simulink model "robotarm_part_both"  (R2018b)
settings: Solver=FixedStepAuto  StartTime=0.0  StopTime=options.T_train-options.dt  RelTol=1e-3  AbsTol=1e-6
undefined symbols (not defined in the file or in its folder): options
libraries: neural x132, simulink x4
(part 2 of 6)

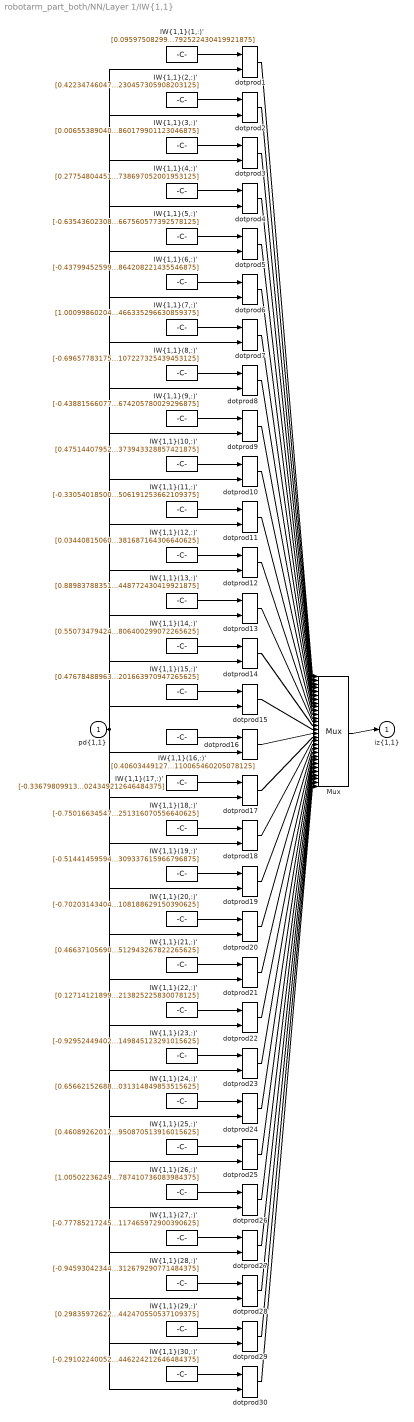
== system robotarm_part_both/NN/Layer 1/IW{1,1} ==
  "pd{1,1}" : Inport  PortDimensions=10
      mask Display: e = 0.06;c1 = [120 230 180]/255;c2 = ([120 230 180]+0)/(256+128);c3 = ([120 230 180]+128)/(256+128);patch([0 1 1 0],[0 0 1 1],c1);patch([0 1 1 1-e 1-e 0+e],[0 0 1 1-e 0+e 0+e],c2);patch([0 0 1 1-e 0+e 0+e],[0 1 1 1-e 1-e 0+e],c3);plot([0 1 1 0 0],[0 0 1 1 0]);
  "IW{1,1}(1,:)'" : Constant  Value=[0.09597508299962474731525929882991476915776729583740234375;0.1005968170649829962481902612125850282609462738037109375;-0.55045262317495780024501073057763278484344482421875;-0.5647944454818947246366178660537116229534149169921875;0.18118548745802998123366478466778062283992767333984375;0.9302020854734853738676747525460086762905120849609375;0.33129531414507751296838478083373047411441802978515625;1.2080937875825370486637666544993408024311065673828125;-0.303614801234934839069268264211132191121578216552734375;-0.64616365051114577067181699021602980792522430419921875]
      mask Display: e = 0.06;c1 = [120 150 230]/255;c2 = ([120 150 230]+0)/383;c3 = ([120 150 230]+128)/383;patch([0 1 1 0],[0 0 1 1],c1);patch([0 1 1 1-e 1-e 0+e],[0 0 1 1-e 0+e 0+e],c2);patch([0 0 1 1-e 0+e 0+e],[0 1 1 1-e 1-e 0+e],c3);plot([0 1 1 0 0],[0 0 1 1 0]);disp('Weights');
  "IW{1,1}(10,:)'" : Constant  Value=[0.47514407952864823325711540746851824223995208740234375;-0.5065631999531381435275534386164508759975433349609375;0.423535188943548301931940613940241746604442596435546875;0.58875725936849587771604319641483016312122344970703125;0.07117432075978487315826015446873498149216175079345703125;-0.5875257273326657259104877084610052406787872314453125;-1.1175178395749139070858291233889758586883544921875;-0.6724331101001104205039382577524520456790924072265625;0.1606137196925800647573367996301385574042797088623046875;-0.0059917862738066256234059636653910274617373943328857421875]
      mask Display: e = 0.06;c1 = [120 150 230]/255;c2 = ([120 150 230]+0)/383;c3 = ([120 150 230]+128)/383;patch([0 1 1 0],[0 0 1 1],c1);patch([0 1 1 1-e 1-e 0+e],[0 0 1 1-e 0+e 0+e],c2);patch([0 0 1 1-e 0+e 0+e],[0 1 1 1-e 1-e 0+e],c3);plot([0 1 1 0 0],[0 0 1 1 0]);disp('Weights');
  "IW{1,1}(11,:)'" : Constant  Value=[-0.330540185002522968193972019435022957623004913330078125;-0.5853737960314406851836110945441760122776031494140625;-0.373973670570021343717570516673731617629528045654296875;-0.457347659514774462774511221141437999904155731201171875;-0.41561353090748831551337616474484093487262725830078125;0.51656871771152046424191439655260182917118072509765625;0.65290213175343636553549231393844820559024810791015625;-0.91601082511943066055692952431854791939258575439453125;-0.414078886006279012210740120281116105616092681884765625;-0.64754463829876518499162330044782720506191253662109375]
      mask Display: e = 0.06;c1 = [120 150 230]/255;c2 = ([120 150 230]+0)/383;c3 = ([120 150 230]+128)/383;patch([0 1 1 0],[0 0 1 1],c1);patch([0 1 1 1-e 1-e 0+e],[0 0 1 1-e 0+e 0+e],c2);patch([0 0 1 1-e 0+e 0+e],[0 1 1 1-e 1-e 0+e],c3);plot([0 1 1 0 0],[0 0 1 1 0]);disp('Weights');
  "IW{1,1}(12,:)'" : Constant  Value=[0.03440815060161195315657778337481431663036346435546875;-0.550528645065602173502838923013769090175628662109375;0.10571613935137315343215647089891717769205570220947265625;-0.50746669530979826578942493142676539719104766845703125;1.216730766600212287897875285125337541103363037109375;0.1123742853737608182740359552553854882717132568359375;-0.66521689864983069018222749946289695799350738525390625;-0.8226026955605025836604227151838131248950958251953125;0.09635653093671248115015259827487170696258544921875;0.92693103311651869891107935472973622381687164306640625]
      mask Display: e = 0.06;c1 = [120 150 230]/255;c2 = ([120 150 230]+0)/383;c3 = ([120 150 230]+128)/383;patch([0 1 1 0],[0 0 1 1],c1);patch([0 1 1 1-e 1-e 0+e],[0 0 1 1-e 0+e 0+e],c2);patch([0 0 1 1-e 0+e 0+e],[0 1 1 1-e 1-e 0+e],c3);plot([0 1 1 0 0],[0 0 1 1 0]);disp('Weights');
  "IW{1,1}(13,:)'" : Constant  Value=[0.889837883519465577819573809392750263214111328125;-0.8578294294074966241936408550827763974666595458984375;-0.50271543951528119276161987727391533553600311279296875;-0.8392445494208258249813070506206713616847991943359375;-0.37185381356888413950656513407011516392230987548828125;0.10486471590851238755437435656858724541962146759033203125;-0.72040207725035998453932961638201959431171417236328125;-0.50713673478396514848753895421396009624004364013671875;-0.1213277153774741379255175388607312925159931182861328125;0.06129702672424190701416790716393734328448772430419921875]
      mask Display: e = 0.06;c1 = [120 150 230]/255;c2 = ([120 150 230]+0)/383;c3 = ([120 150 230]+128)/383;patch([0 1 1 0],[0 0 1 1],c1);patch([0 1 1 1-e 1-e 0+e],[0 0 1 1-e 0+e 0+e],c2);patch([0 0 1 1-e 0+e 0+e],[0 1 1 1-e 1-e 0+e],c3);plot([0 1 1 0 0],[0 0 1 1 0]);disp('Weights');
  "IW{1,1}(14,:)'" : Constant  Value=[0.550734794240352432126428539049811661243438720703125;0.053975292722394645206218655175689491443336009979248046875;1.212308009175175005367464109440334141254425048828125;-0.39026739480771788226576290981029160320758819580078125;-0.30993818648640125701376746292226016521453857421875;0.230175159246569116522351805542712099850177764892578125;-0.2396188690138271459861840639860020019114017486572265625;0.46962187422249479507030400782241486012935638427734375;-0.64883949282064889985122135840356349945068359375;0.749542964618973517332278788671828806400299072265625]
      mask Display: e = 0.06;c1 = [120 150 230]/255;c2 = ([120 150 230]+0)/383;c3 = ([120 150 230]+128)/383;patch([0 1 1 0],[0 0 1 1],c1);patch([0 1 1 1-e 1-e 0+e],[0 0 1 1-e 0+e 0+e],c2);patch([0 0 1 1-e 0+e 0+e],[0 1 1 1-e 1-e 0+e],c3);plot([0 1 1 0 0],[0 0 1 1 0]);disp('Weights');
  "IW{1,1}(15,:)'" : Constant  Value=[0.476784889630048114295135519569157622754573822021484375;-1.1575538515421330831856039367266930639743804931640625;0.74998910290864151395595627036527730524539947509765625;0.686868502075232978398844352341257035732269287109375;0.55518939608199147084377500505070202052593231201171875;-0.180624972118895221750989321662927977740764617919921875;0.675483264307952691041236903402023017406463623046875;-0.1325719972276437896852030462468974292278289794921875;0.33056839807348759041616403919761069118976593017578125;-0.43316098724255402974137041383073665201663970947265625]
      mask Display: e = 0.06;c1 = [120 150 230]/255;c2 = ([120 150 230]+0)/383;c3 = ([120 150 230]+128)/383;patch([0 1 1 0],[0 0 1 1],c1);patch([0 1 1 1-e 1-e 0+e],[0 0 1 1-e 0+e 0+e],c2);patch([0 0 1 1-e 0+e 0+e],[0 1 1 1-e 1-e 0+e],c3);plot([0 1 1 0 0],[0 0 1 1 0]);disp('Weights');
  "IW{1,1}(16,:)'" : Constant  Value=[0.406034491279999854018711857861489988863468170166015625;-0.56064208448016195074359302452648989856243133544921875;0.312057743964170797301704851633985526859760284423828125;-0.941004166867964730869289269321598112583160400390625;0.1376339095606373963409652105838176794350147247314453125;0.67401897919977837858596103615127503871917724609375;0.550579076991224436454785973182879388332366943359375;-0.64279023731962769971914894995279610157012939453125;-0.8904111453933516440173434602911584079265594482421875;0.003560833561972812262574894504041367326863110065460205078125]
      mask Display: e = 0.06;c1 = [120 150 230]/255;c2 = ([120 150 230]+0)/383;c3 = ([120 150 230]+128)/383;patch([0 1 1 0],[0 0 1 1],c1);patch([0 1 1 1-e 1-e 0+e],[0 0 1 1-e 0+e 0+e],c2);patch([0 0 1 1-e 0+e 0+e],[0 1 1 1-e 1-e 0+e],c3);plot([0 1 1 0 0],[0 0 1 1 0]);disp('Weights');
  "IW{1,1}(17,:)'" : Constant  Value=[-0.33679809913795033526895394970779307186603546142578125;-0.36043707070088937260976535981171764433383941650390625;-0.0935795546537070699333327183921937830746173858642578125;0.731185172321640042270018966519273817539215087890625;-0.5718811855197476479162332907435484230518341064453125;0.84242307124785165139968512448831461369991302490234375;0.95733279790061509562093533531879074871540069580078125;0.65303929509592162361286682425998151302337646484375;-0.314864426487880877392200318354298360645771026611328125;-0.330246746774365274035289985476993024349212646484375]
      mask Display: e = 0.06;c1 = [120 150 230]/255;c2 = ([120 150 230]+0)/383;c3 = ([120 150 230]+128)/383;patch([0 1 1 0],[0 0 1 1],c1);patch([0 1 1 1-e 1-e 0+e],[0 0 1 1-e 0+e 0+e],c2);patch([0 0 1 1-e 0+e 0+e],[0 1 1 1-e 1-e 0+e],c3);plot([0 1 1 0 0],[0 0 1 1 0]);disp('Weights');
  "IW{1,1}(18,:)'" : Constant  Value=[-0.7501663454733940028518190956674516201019287109375;-0.754548594542325812284389030537568032741546630859375;0.37038472779503461840278077943366952240467071533203125;-0.1562935424990742061535087259471765719354152679443359375;0.138543467118524110670563231906271539628505706787109375;0.29325556026231580641905338779906742274761199951171875;0.5557533987560876465039427785086445510387420654296875;-0.5891598679021805562427971381112001836299896240234375;0.93703964326763011793985924668959341943264007568359375;0.9411371236734513701094329007901251316070556640625]
      mask Display: e = 0.06;c1 = [120 150 230]/255;c2 = ([120 150 230]+0)/383;c3 = ([120 150 230]+128)/383;patch([0 1 1 0],[0 0 1 1],c1);patch([0 1 1 1-e 1-e 0+e],[0 0 1 1-e 0+e 0+e],c2);patch([0 0 1 1-e 0+e 0+e],[0 1 1 1-e 1-e 0+e],c3);plot([0 1 1 0 0],[0 0 1 1 0]);disp('Weights');
  "IW{1,1}(19,:)'" : Constant  Value=[-0.51441459594363536655947655162890441715717315673828125;0.9898609829948823435330496067763306200504302978515625;-0.1761918696090294667033759878904675133526325225830078125;0.7054084177556150248022959203808568418025970458984375;1.1060012216382795191549348601256497204303741455078125;-0.41983895450718089481512151905917562544345855712890625;-0.47814762490560080987478386305156163871288299560546875;0.09572687926285235182621846661277231760323047637939453125;-0.63750175599319069963399897460476495325565338134765625;-0.60128781969086009251412860976415686309337615966796875]
      mask Display: e = 0.06;c1 = [120 150 230]/255;c2 = ([120 150 230]+0)/383;c3 = ([120 150 230]+128)/383;patch([0 1 1 0],[0 0 1 1],c1);patch([0 1 1 1-e 1-e 0+e],[0 0 1 1-e 0+e 0+e],c2);patch([0 0 1 1-e 0+e 0+e],[0 1 1 1-e 1-e 0+e],c3);plot([0 1 1 0 0],[0 0 1 1 0]);disp('Weights');
  "IW{1,1}(2,:)'" : Constant  Value=[0.4223474604711616731123058343655429780483245849609375;-0.2554232271341405624553999587078578770160675048828125;-0.675779357385505097255418149870820343494415283203125;0.283625216190791729076181582058779895305633544921875;-0.143599144624300734118804712124983780086040496826171875;-0.5893666969145778811167701860540546476840972900390625;1.028076357601400037111716301296837627887725830078125;-0.70744355393608004956007562213926576077938079833984375;-0.83454591678897360740307931337156333029270172119140625;-0.70479890544089596193799707180005498230457305908203125]
      mask Display: e = 0.06;c1 = [120 150 230]/255;c2 = ([120 150 230]+0)/383;c3 = ([120 150 230]+128)/383;patch([0 1 1 0],[0 0 1 1],c1);patch([0 1 1 1-e 1-e 0+e],[0 0 1 1-e 0+e 0+e],c2);patch([0 0 1 1-e 0+e 0+e],[0 1 1 1-e 1-e 0+e],c3);plot([0 1 1 0 0],[0 0 1 1 0]);disp('Weights');
  "IW{1,1}(20,:)'" : Constant  Value=[-0.7020314340426152543983562281937338411808013916015625;0.374747170887574865272284796446911059319972991943359375;0.80256243474079724808945002223481424152851104736328125;0.92052377567109500144937328514060936868190765380859375;-0.56430728708136179694321299393777735531330108642578125;-0.409268793962840049527329711054335348308086395263671875;-0.63522912877429049682831418977002613246440887451171875;0.749757753512940272599962554522790014743804931640625;-0.242439340225094224212654125949484296143054962158203125;-0.62137271108860370194548750077956356108188629150390625]
      mask Display: e = 0.06;c1 = [120 150 230]/255;c2 = ([120 150 230]+0)/383;c3 = ([120 150 230]+128)/383;patch([0 1 1 0],[0 0 1 1],c1);patch([0 1 1 1-e 1-e 0+e],[0 0 1 1-e 0+e 0+e],c2);patch([0 0 1 1-e 0+e 0+e],[0 1 1 1-e 1-e 0+e],c3);plot([0 1 1 0 0],[0 0 1 1 0]);disp('Weights');
  "IW{1,1}(21,:)'" : Constant  Value=[0.466371056901808744843407339430996216833591461181640625;0.23923374353719373264226533137843944132328033447265625;-0.502233468102315949721514698467217385768890380859375;1.0295964740352392396971481502987444400787353515625;-0.75326351082972620165634225486428476870059967041015625;0.635138525967285705320364286308176815509796142578125;0.88613675552031312410150576397427357733249664306640625;0.2011640793059821519239704912251909263432025909423828125;0.7478976029053165941462566479458473622798919677734375;0.058977656358513631806861354789361939765512943267822265625]
      mask Display: e = 0.06;c1 = [120 150 230]/255;c2 = ([120 150 230]+0)/383;c3 = ([120 150 230]+128)/383;patch([0 1 1 0],[0 0 1 1],c1);patch([0 1 1 1-e 1-e 0+e],[0 0 1 1-e 0+e 0+e],c2);patch([0 0 1 1-e 0+e 0+e],[0 1 1 1-e 1-e 0+e],c3);plot([0 1 1 0 0],[0 0 1 1 0]);disp('Weights');
  "IW{1,1}(22,:)'" : Constant  Value=[0.1271412189932890901555850859949714504182338714599609375;-0.1379965584445177473327248662826605141162872314453125;0.72963482668915491391459227088489569723606109619140625;-0.71766209204583863989768133251345716416835784912109375;0.7607687121077024716697678741184063255786895751953125;-0.9611143517657279033983286353759467601776123046875;-0.80962560893681345675076954648829996585845947265625;0.63315517539712862227219147825962863862514495849609375;0.005627955669525182280654718169898842461407184600830078125;-0.402668774031742338070927189619396813213825225830078125]
      mask Display: e = 0.06;c1 = [120 150 230]/255;c2 = ([120 150 230]+0)/383;c3 = ([120 150 230]+128)/383;patch([0 1 1 0],[0 0 1 1],c1);patch([0 1 1 1-e 1-e 0+e],[0 0 1 1-e 0+e 0+e],c2);patch([0 0 1 1-e 0+e 0+e],[0 1 1 1-e 1-e 0+e],c3);plot([0 1 1 0 0],[0 0 1 1 0]);disp('Weights');
  "IW{1,1}(23,:)'" : Constant  Value=[-0.92952449402361647656789500615559518337249755859375;-0.0211037669750557300984983299940722645260393619537353515625;0.048135582502047725983462811427671113051474094390869140625;0.50922777724496592899328106796019710600376129150390625;-0.50732495978172031936281882735784165561199188232421875;-0.69676951843595447133594689148594625294208526611328125;-0.65547410734391409192767241620458662509918212890625;-0.0014210247511794627146841651921249649603851139545440673828125;-0.868827381912322227464073876035399734973907470703125;-0.67155869735658824115631659878999926149845123291015625]
      mask Display: e = 0.06;c1 = [120 150 230]/255;c2 = ([120 150 230]+0)/383;c3 = ([120 150 230]+128)/383;patch([0 1 1 0],[0 0 1 1],c1);patch([0 1 1 1-e 1-e 0+e],[0 0 1 1-e 0+e 0+e],c2);patch([0 0 1 1-e 0+e 0+e],[0 1 1 1-e 1-e 0+e],c3);plot([0 1 1 0 0],[0 0 1 1 0]);disp('Weights');
  "IW{1,1}(24,:)'" : Constant  Value=[0.6566215268892212630902349701500497758388519287109375;0.35191303857450961789510301969130523502826690673828125;0.0887872045633903705930123351208749227225780487060546875;-0.52167538237939492518080442096106708049774169921875;-0.81772280753968351607596787289367057383060455322265625;-0.486116058291732766605264259851537644863128662109375;0.02923370252754010911733217881192103959619998931884765625;0.65606898533962676456354756737709976732730865478515625;1.069510188925867577580675060744397342205047607421875;-0.349587636209095775630117941545904614031314849853515625]
      mask Display: e = 0.06;c1 = [120 150 230]/255;c2 = ([120 150 230]+0)/383;c3 = ([120 150 230]+128)/383;patch([0 1 1 0],[0 0 1 1],c1);patch([0 1 1 1-e 1-e 0+e],[0 0 1 1-e 0+e 0+e],c2);patch([0 0 1 1-e 0+e 0+e],[0 1 1 1-e 1-e 0+e],c3);plot([0 1 1 0 0],[0 0 1 1 0]);disp('Weights');
  "IW{1,1}(25,:)'" : Constant  Value=[0.460892620125363972061194317575427703559398651123046875;-0.702983849519208892075994299375452101230621337890625;0.71961841332974063600858016798156313598155975341796875;0.169022484457222288423139389124116860330104827880859375;0.705019672467758429235118455835618078708648681640625;0.9106824677630818154483449688996188342571258544921875;-0.78555018806189291780128769460134208202362060546875;0.07855809248696388191746109441737644374370574951171875;-0.518148513136680310964266027440316975116729736328125;0.33595115214708271000887407353729940950870513916015625]
      mask Display: e = 0.06;c1 = [120 150 230]/255;c2 = ([120 150 230]+0)/383;c3 = ([120 150 230]+128)/383;patch([0 1 1 0],[0 0 1 1],c1);patch([0 1 1 1-e 1-e 0+e],[0 0 1 1-e 0+e 0+e],c2);patch([0 0 1 1-e 0+e 0+e],[0 1 1 1-e 1-e 0+e],c3);plot([0 1 1 0 0],[0 0 1 1 0]);disp('Weights');
  "IW{1,1}(26,:)'" : Constant  Value=[1.0050223624965364255245958702289499342441558837890625;-0.80488037773500342719756872611469589173793792724609375;-0.5427477332576418067588974736281670629978179931640625;-0.56695170645189574276656685469788499176502227783203125;0.8180594878356888255410694910096935927867889404296875;0.54460022333480484491019524284638464450836181640625;-0.55968520956281297973333721529343165457248687744140625;-0.42491469834192419074980762161430902779102325439453125;-0.181225284991976598458762737209326587617397308349609375;0.01952552575827526393226207801490090787410736083984375]
      mask Display: e = 0.06;c1 = [120 150 230]/255;c2 = ([120 150 230]+0)/383;c3 = ([120 150 230]+128)/383;patch([0 1 1 0],[0 0 1 1],c1);patch([0 1 1 1-e 1-e 0+e],[0 0 1 1-e 0+e 0+e],c2);patch([0 0 1 1-e 0+e 0+e],[0 1 1 1-e 1-e 0+e],c3);plot([0 1 1 0 0],[0 0 1 1 0]);disp('Weights');
  "IW{1,1}(27,:)'" : Constant  Value=[-0.777852172459911894719652991625480353832244873046875;-0.9628992337469119977555465084151364862918853759765625;0.97490019983532050229513288286398164927959442138671875;-0.00514387590413110419584885590893463813699781894683837890625;0.176157855600243939964144601617590524256229400634765625;0.130275262732087060424390756452339701354503631591796875;-0.68732090121583222508405697226407937705516815185546875;0.6813542353846659960225906615960411727428436279296875;0.260914856848821707924201973582967184484004974365234375;-0.3877040493921521946418806692236103117465972900390625]
      mask Display: e = 0.06;c1 = [120 150 230]/255;c2 = ([120 150 230]+0)/383;c3 = ([120 150 230]+128)/383;patch([0 1 1 0],[0 0 1 1],c1);patch([0 1 1 1-e 1-e 0+e],[0 0 1 1-e 0+e 0+e],c2);patch([0 0 1 1-e 0+e 0+e],[0 1 1 1-e 1-e 0+e],c3);plot([0 1 1 0 0],[0 0 1 1 0]);disp('Weights');
  "IW{1,1}(28,:)'" : Constant  Value=[-0.9459304234482968087860399464261718094348907470703125;0.6511299391851366191730221544275991618633270263671875;-0.296631290162832683687810231276671402156352996826171875;0.0661545673622102314848092419197200797498226165771484375;0.089346572239912658286442592725506983697414398193359375;-1.2788532682797859596490752664976753294467926025390625;0.700141465610315538725672013242729008197784423828125;-0.0935827563477613366682561490961234085261821746826171875;0.207675198151261841683634656874346546828746795654296875;-0.07307146341374336218077445437302230857312679290771484375]
      mask Display: e = 0.06;c1 = [120 150 230]/255;c2 = ([120 150 230]+0)/383;c3 = ([120 150 230]+128)/383;patch([0 1 1 0],[0 0 1 1],c1);patch([0 1 1 1-e 1-e 0+e],[0 0 1 1-e 0+e 0+e],c2);patch([0 0 1 1-e 0+e 0+e],[0 1 1 1-e 1-e 0+e],c3);plot([0 1 1 0 0],[0 0 1 1 0]);disp('Weights');
  "IW{1,1}(29,:)'" : Constant  Value=[0.298359726225109922470579704167903400957584381103515625;-0.396701786335596773280798288396908901631832122802734375;-1.13370657543820474444373758160509169101715087890625;-0.2805861564483913550560600924654863774776458740234375;0.4696583031682493025726898849825374782085418701171875;1.0702946811240254820773998289951123297214508056640625;0.28248447024084766265872303847572766244411468505859375;-0.062823106516774973595573783313739113509654998779296875;-0.24131048284781375645735579382744617760181427001953125;0.8034308293115477450641037648892961442470550537109375]
      mask Display: e = 0.06;c1 = [120 150 230]/255;c2 = ([120 150 230]+0)/383;c3 = ([120 150 230]+128)/383;patch([0 1 1 0],[0 0 1 1],c1);patch([0 1 1 1-e 1-e 0+e],[0 0 1 1-e 0+e 0+e],c2);patch([0 0 1 1-e 0+e 0+e],[0 1 1 1-e 1-e 0+e],c3);plot([0 1 1 0 0],[0 0 1 1 0]);disp('Weights');
  "IW{1,1}(3,:)'" : Constant  Value=[0.00655389040905785848212250499500441947020590305328369140625;-0.6045148029370317477315666110371239483356475830078125;-0.476254697613530952882143765236833132803440093994140625;0.63520112506088233228496164883836172521114349365234375;-0.62319560772153181904542407210101373493671417236328125;-0.66765899625154501162427322924486361443996429443359375;0.87911400831377528586330072357668541371822357177734375;0.42374944665044378400153846087050624191761016845703125;-0.439816857191326848752765954486676491796970367431640625;-0.97754507101669385615849705573054961860179901123046875]
      mask Display: e = 0.06;c1 = [120 150 230]/255;c2 = ([120 150 230]+0)/383;c3 = ([120 150 230]+128)/383;patch([0 1 1 0],[0 0 1 1],c1);patch([0 1 1 1-e 1-e 0+e],[0 0 1 1-e 0+e 0+e],c2);patch([0 0 1 1-e 0+e 0+e],[0 1 1 1-e 1-e 0+e],c3);plot([0 1 1 0 0],[0 0 1 1 0]);disp('Weights');
  "IW{1,1}(30,:)'" : Constant  Value=[-0.291022400523337498867704198346473276615142822265625;0.580625810949982668063285018433816730976104736328125;0.19536375184446763686452186448150314390659332275390625;0.64964684143537265725854012998752295970916748046875;0.76038407040179567530913118389435112476348876953125;-0.05098651696890361961767013099233736284077167510986328125;-0.252987456128652699050007868208922445774078369140625;0.92036050173776373650724735853145830333232879638671875;0.98871167709859564265428844009875319898128509521484375;-0.2278183219186088181995586410266696475446224212646484375]
      mask Display: e = 0.06;c1 = [120 150 230]/255;c2 = ([120 150 230]+0)/383;c3 = ([120 150 230]+128)/383;patch([0 1 1 0],[0 0 1 1],c1);patch([0 1 1 1-e 1-e 0+e],[0 0 1 1-e 0+e 0+e],c2);patch([0 0 1 1-e 0+e 0+e],[0 1 1 1-e 1-e 0+e],c3);plot([0 1 1 0 0],[0 0 1 1 0]);disp('Weights');
  "IW{1,1}(4,:)'" : Constant  Value=[0.277548044517540282161149889361695386469364166259765625;0.37749232938269716708390433268505148589611053466796875;0.078289089815219037316040839868946932256221771240234375;0.98855009632125201424202032285393215715885162353515625;-0.14164230747110340136174500003107823431491851806640625;-0.9366218154343339818979075062088668346405029296875;-0.484206406521606458337458889218396507203578948974609375;-0.04090898418104427225472363716107793152332305908203125;-1.0727071601977720138876293276553042232990264892578125;0.259646897113359476083616073083248920738697052001953125]
      mask Display: e = 0.06;c1 = [120 150 230]/255;c2 = ([120 150 230]+0)/383;c3 = ([120 150 230]+128)/383;patch([0 1 1 0],[0 0 1 1],c1);patch([0 1 1 1-e 1-e 0+e],[0 0 1 1-e 0+e 0+e],c2);patch([0 0 1 1-e 0+e 0+e],[0 1 1 1-e 1-e 0+e],c3);plot([0 1 1 0 0],[0 0 1 1 0]);disp('Weights');
  "IW{1,1}(5,:)'" : Constant  Value=[-0.63543602308178959159334908690652810037136077880859375;0.4879055831469985005099943009554408490657806396484375;0.08173822552504152183505681250608176924288272857666015625;-0.83340546323539010931114034974598325788974761962890625;-0.7207066141016558180609763439861126244068145751953125;-0.58539429529925557371683453311561606824398040771484375;-0.4712133145390222654924627931904979050159454345703125;0.08514951952846515348394262900910689495503902435302734375;0.41653833109728799488635786474333144724369049072265625;0.88711189581884675181555621747975237667560577392578125]
      mask Display: e = 0.06;c1 = [120 150 230]/255;c2 = ([120 150 230]+0)/383;c3 = ([120 150 230]+128)/383;patch([0 1 1 0],[0 0 1 1],c1);patch([0 1 1 1-e 1-e 0+e],[0 0 1 1-e 0+e 0+e],c2);patch([0 0 1 1-e 0+e 0+e],[0 1 1 1-e 1-e 0+e],c3);plot([0 1 1 0 0],[0 0 1 1 0]);disp('Weights');
  "IW{1,1}(6,:)'" : Constant  Value=[-0.437994525994974515104019019418046809732913970947265625;-0.324878219388466227268708053088630549609661102294921875;-0.83601690351700785885924460671958513557910919189453125;0.48177266852916622585922823418513871729373931884765625;-0.61727856845805917362923764812876470386981964111328125;0.9678446003847589462765199641580693423748016357421875;0.80952515780822498214774896041490137577056884765625;-0.326304649280063141514318658664706163108348846435546875;0.50218510820433837071874449975439347326755523681640625;0.114370243600563081809440291181090287864208221435546875]
      mask Display: e = 0.06;c1 = [120 150 230]/255;c2 = ([120 150 230]+0)/383;c3 = ([120 150 230]+128)/383;patch([0 1 1 0],[0 0 1 1],c1);patch([0 1 1 1-e 1-e 0+e],[0 0 1 1-e 0+e 0+e],c2);patch([0 0 1 1-e 0+e 0+e],[0 1 1 1-e 1-e 0+e],c3);plot([0 1 1 0 0],[0 0 1 1 0]);disp('Weights');
  "IW{1,1}(7,:)'" : Constant  Value=[1.0009986020461105749035368717159144580364227294921875;-1.08238337452271249361501759267412126064300537109375;-0.034163425622081820820508113456526189111173152923583984375;-0.024211618185480753007166043744291528128087520599365234375;-0.61405766995675870045801048036082647740840911865234375;-0.491690139481823218492451132988207973539829254150390625;-0.00522869761890705497808795598757569678127765655517578125;0.389808867986846274700241110622300766408443450927734375;-0.9572685474589501808395652915351092815399169921875;-0.42426148597732049605468773734173737466335296630859375]
      mask Display: e = 0.06;c1 = [120 150 230]/255;c2 = ([120 150 230]+0)/383;c3 = ([120 150 230]+128)/383;patch([0 1 1 0],[0 0 1 1],c1);patch([0 1 1 1-e 1-e 0+e],[0 0 1 1-e 0+e 0+e],c2);patch([0 0 1 1-e 0+e 0+e],[0 1 1 1-e 1-e 0+e],c3);plot([0 1 1 0 0],[0 0 1 1 0]);disp('Weights');
  "IW{1,1}(8,:)'" : Constant  Value=[-0.696577831755603060770454248995520174503326416015625;0.260928819297299663393374657971435226500034332275390625;-0.222129775732852419167784319142811000347137451171875;0.83862169652570861533291690648184157907962799072265625;-0.93426204340168428341684148108470253646373748779296875;0.59728809042987573985072913274052552878856658935546875;-0.205824792521768384911950988680473528802394866943359375;-0.351510023204236798921584750132751651108264923095703125;-0.8082537928258499704270434449426829814910888671875;0.490225662549016949487423744358238764107227325439453125]
      mask Display: e = 0.06;c1 = [120 150 230]/255;c2 = ([120 150 230]+0)/383;c3 = ([120 150 230]+128)/383;patch([0 1 1 0],[0 0 1 1],c1);patch([0 1 1 1-e 1-e 0+e],[0 0 1 1-e 0+e 0+e],c2);patch([0 0 1 1-e 0+e 0+e],[0 1 1 1-e 1-e 0+e],c3);plot([0 1 1 0 0],[0 0 1 1 0]);disp('Weights');
  "IW{1,1}(9,:)'" : Constant  Value=[-0.438815660773629379054483479194459505379199981689453125;0.022995226860754384989871113020853954367339611053466796875;-0.78080728835096768758461394099867902696132659912109375;-0.80299424756420012538882247099536471068859100341796875;-0.45808703980880849382373298794846050441265106201171875;0.58467027085579237333234914331114850938320159912109375;0.7156103557142385884759505643160082399845123291015625;-0.9261791543164930029519155141315422952175140380859375;0.348270725250001189632342857294133864343166351318359375;-0.3221259786675698677527179825119674205780029296875]
      mask Display: e = 0.06;c1 = [120 150 230]/255;c2 = ([120 150 230]+0)/383;c3 = ([120 150 230]+128)/383;patch([0 1 1 0],[0 0 1 1],c1);patch([0 1 1 1-e 1-e 0+e],[0 0 1 1-e 0+e 0+e],c2);patch([0 0 1 1-e 0+e 0+e],[0 1 1 1-e 1-e 0+e],c3);plot([0 1 1 0 0],[0 0 1 1 0]);disp('Weights');
  Mux : Mux  Inputs=30
      mask Display: e = 0.06;c1 = [120 150 230]/255;c2 = ([120 150 230]+0)/383;c3 = ([120 150 230]+128)/383;patch([0 1 1 0],[0 0 1 1],c1);patch([0 1 1 1-e 1-e 0+e],[0 0 1 1-e 0+e 0+e],c2);patch([0 0 1 1-e 0+e 0+e],[0 1 1 1-e 1-e 0+e],c3);plot([0 1 1 0 0],[0 0 1 1 0]);disp('Mux');
  dotprod{1..30} (30 alike) : neural/Weight Functions/dotprod
  "iz{1,1}" : Outport
      mask Display: e = 0.06;c1 = [120 230 180]/255;c2 = ([120 230 180]+0)/(256+128);c3 = ([120 230 180]+128)/(256+128);patch([0 1 1 0],[0 0 1 1],c1);patch([0 1 1 1-e 1-e 0+e],[0 0 1 1-e 0+e 0+e],c2);patch([0 0 1 1-e 0+e 0+e],[0 1 1 1-e 1-e 0+e],c3);plot([0 1 1 0 0],[0 0 1 1 0]);
  wires:
  "IW{1,1}(1,:)'"/1 -> dotprod1/1
  "pd{1,1}"/1 -> dotprod1/2, dotprod2/2, dotprod3/2, dotprod4/2, dotprod5/2, dotprod6/2, dotprod7/2, dotprod8/2, dotprod9/2, dotprod10/2, dotprod11/2, dotprod12/2, dotprod13/2, dotprod14/2, dotprod15/2, dotprod16/2, dotprod17/2, dotprod18/2, dotprod19/2, dotprod20/2, dotprod21/2, dotprod22/2, dotprod23/2, dotprod24/2, dotprod25/2, dotprod26/2, dotprod27/2, dotprod28/2, dotprod29/2, dotprod30/2
  dotprod1/1 -> Mux/1
  "IW{1,1}(2,:)'"/1 -> dotprod2/1
  dotprod2/1 -> Mux/2
  "IW{1,1}(3,:)'"/1 -> dotprod3/1
  dotprod3/1 -> Mux/3
  "IW{1,1}(4,:)'"/1 -> dotprod4/1
  dotprod4/1 -> Mux/4
  "IW{1,1}(5,:)'"/1 -> dotprod5/1
  dotprod5/1 -> Mux/5
  "IW{1,1}(6,:)'"/1 -> dotprod6/1
  dotprod6/1 -> Mux/6
  "IW{1,1}(7,:)'"/1 -> dotprod7/1
  dotprod7/1 -> Mux/7
  "IW{1,1}(8,:)'"/1 -> dotprod8/1
  dotprod8/1 -> Mux/8
  "IW{1,1}(9,:)'"/1 -> dotprod9/1
  dotprod9/1 -> Mux/9
  "IW{1,1}(10,:)'"/1 -> dotprod10/1
  dotprod10/1 -> Mux/10
  "IW{1,1}(11,:)'"/1 -> dotprod11/1
  dotprod11/1 -> Mux/11
  "IW{1,1}(12,:)'"/1 -> dotprod12/1
  dotprod12/1 -> Mux/12
  "IW{1,1}(13,:)'"/1 -> dotprod13/1
  dotprod13/1 -> Mux/13
  "IW{1,1}(14,:)'"/1 -> dotprod14/1
  dotprod14/1 -> Mux/14
  "IW{1,1}(15,:)'"/1 -> dotprod15/1
  dotprod15/1 -> Mux/15
  "IW{1,1}(16,:)'"/1 -> dotprod16/1
  dotprod16/1 -> Mux/16
  "IW{1,1}(17,:)'"/1 -> dotprod17/1
  dotprod17/1 -> Mux/17
  "IW{1,1}(18,:)'"/1 -> dotprod18/1
  dotprod18/1 -> Mux/18
  "IW{1,1}(19,:)'"/1 -> dotprod19/1
  dotprod19/1 -> Mux/19
  "IW{1,1}(20,:)'"/1 -> dotprod20/1
  dotprod20/1 -> Mux/20
  "IW{1,1}(21,:)'"/1 -> dotprod21/1
  dotprod21/1 -> Mux/21
  "IW{1,1}(22,:)'"/1 -> dotprod22/1
  dotprod22/1 -> Mux/22
  "IW{1,1}(23,:)'"/1 -> dotprod23/1
  dotprod23/1 -> Mux/23
  "IW{1,1}(24,:)'"/1 -> dotprod24/1
  dotprod24/1 -> Mux/24
  "IW{1,1}(25,:)'"/1 -> dotprod25/1
  dotprod25/1 -> Mux/25
  "IW{1,1}(26,:)'"/1 -> dotprod26/1
  dotprod26/1 -> Mux/26
  "IW{1,1}(27,:)'"/1 -> dotprod27/1
  dotprod27/1 -> Mux/27
  "IW{1,1}(28,:)'"/1 -> dotprod28/1
  dotprod28/1 -> Mux/28
  "IW{1,1}(29,:)'"/1 -> dotprod29/1
  dotprod29/1 -> Mux/29
  "IW{1,1}(30,:)'"/1 -> dotprod30/1
  dotprod30/1 -> Mux/30
  Mux/1 -> "iz{1,1}"/1

== system robotarm_part_both/NN/Layer 2/Delays 1 ==
  "p{2}" : Inport  PortDimensions=30
      mask Display: e = 0.06;c1 = [120 230 180]/255;c2 = ([120 230 180]+0)/(256+128);c3 = ([120 230 180]+128)/(256+128);patch([0 1 1 0],[0 0 1 1],c1);patch([0 1 1 1-e 1-e 0+e],[0 0 1 1-e 0+e 0+e],c2);patch([0 0 1 1-e 0+e 0+e],[0 1 1 1-e 1-e 0+e],c3);plot([0 1 1 0 0],[0 0 1 1 0]);
  mux : Mux  Inputs=1
      mask Display: e = 0.06;c1 = [120 150 230]/255;c2 = ([120 150 230]+0)/383;c3 = ([120 150 230]+128)/383;patch([0 1 1 0],[0 0 1 1],c1);patch([0 1 1 1-e 1-e 0+e],[0 0 1 1-e 0+e 0+e],c2);patch([0 0 1 1-e 0+e 0+e],[0 1 1 1-e 1-e 0+e],c3);plot([0 1 1 0 0],[0 0 1 1 0]);disp('Mux')
  "pd{2,1}" : Outport
      mask Display: e = 0.06;c1 = [120 230 180]/255;c2 = ([120 230 180]+0)/(256+128);c3 = ([120 230 180]+128)/(256+128);patch([0 1 1 0],[0 0 1 1],c1);patch([0 1 1 1-e 1-e 0+e],[0 0 1 1-e 0+e 0+e],c2);patch([0 0 1 1-e 0+e 0+e],[0 1 1 1-e 1-e 0+e],c3);plot([0 1 1 0 0],[0 0 1 1 0]);
  wires:
  "p{2}"/1 -> mux/1
  mux/1 -> "pd{2,1}"/1
